simulink library "Linkage_Systems"  (R2024a)
settings: Solver=VariableStepAuto  StartTime=0.0  StopTime=10.0  RelTol=1e-3
undefined symbols (not defined in the file): Init, Vehicle
libraries: Linkage_DW_B x1, Linkage_DW_Pullrod x1, Linkage_DW_Pullrod_NoSteer x1, Linkage_DW_Pushrod x1, Linkage_DW_Pushrod_NoSteer x1, Linkage_DW_A x1, Linkage_Link5C_S2LAF x1, Linkage_Link5_S2LAC_AU_NoSteer x1, Linkage_Link5_S2LAF x1, Linkage_Link5_S2LAR x1, Linkage_MacPherson x1, Linkage_MacPherson_SpLA x1
(part 2 of 2)

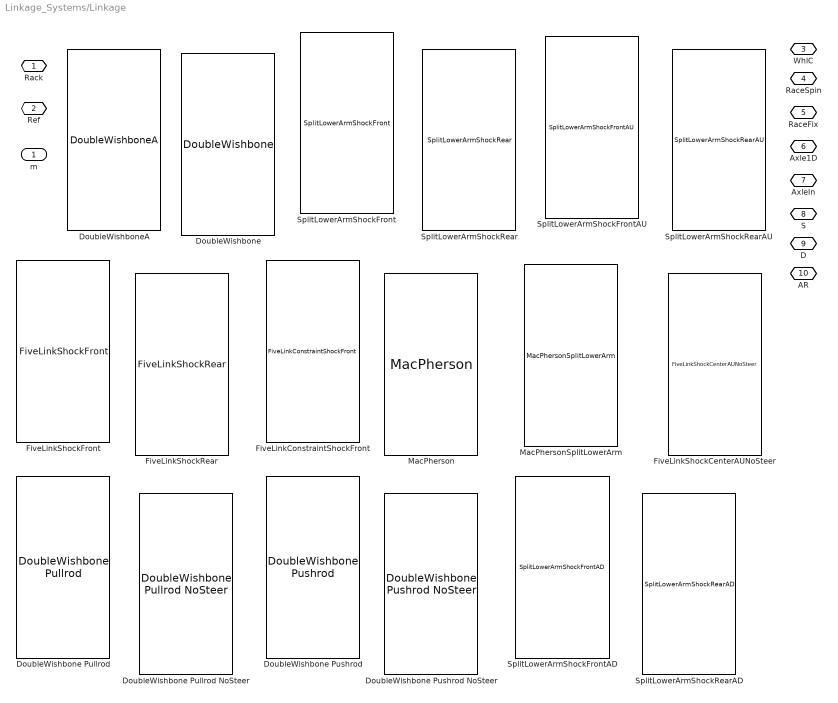
== system Linkage_Systems/Linkage ==
  DoubleWishbone : Linkage_DW_B/DoubleWishbone  VariantControl=DoubleWishbone  popup_leftRight=Left  hp_in_f_ua=Linkage.UpperWishbone.sInboardF.Value  hp_in_r_ua=Linkage.UpperWishbone.sInboardR.Value  hp_out_ua=Linkage.UpperWishbone.sOutboard.Value  hp_in_f_la=Linkage.LowerWishbone.sInboardF.Value  hp_in_r_la=Linkage.LowerWishbone.sInboardR.Value  hp_out_la=Linkage.LowerWishbone.sOutboard.Value  hp_arb=Linkage.LowerWishbone.sARB.Value  hp_upr_cg=Linkage.Upright.sCG.Value  hp_upr_wc=Linkage.Upright.sWheelCentre.Value  hp_in_rod=Linkage.TrackRod.sInboard.Value  hp_upr_rod=Linkage.TrackRod.sOutboard.Value  hp_spr_top=Linkage.Shock.sTop.Value  hp_spr_bot=Linkage.Shock.sBottom.Value  clr_hp=Visual.hp.clr  opc_hp=Visual.hp.opc  size_hp=Visual.hp.rad  Upper_Arm_to_Subframe=Linkage.Upper_Arm_to_Subframe  ua_mass=Linkage.UpperWishbone.m.Value  clr_ua=Visual.UpperArm.clr  opc_ua=Visual.part.opc  radius_ua=Visual.UpperArm.rad  Lower_Arm_to_Subframe=Linkage.Lower_Arm_to_Subframe  arm_mass=Linkage.LowerWishbone.m.Value  clr_la=Visual.LowerArm.clr  opc_la=Visual.part.opc  radius_la=Visual.LowerArm.rad  shock_pist_mass=Linkage.Shock.mPiston.Value  shock_cyl_mass=Linkage.Shock.mCylinder.Value  up_lim_bumpstop=Linkage.Endstop.xMax.Value  low_lim_bumpstop=Linkage.Endstop.xMin.Value  clr_conn_shock=Visual.hp.clr  opc_conn_shock=Visual.hp.opc  size_conn_shock=Visual.hp.rad  clr_shock_cyl=Visual.Shock.cyl.clr  opc_shock_cyl=Visual.part.opc  radius_shock_cyl=Visual.Shock.cyl.rad  clr_shock_piston=Visual.Shock.piston.clr  opc_shock_piston=Visual.part.opc  clr_shock_bumpstop=Visual.Shock.bumpstop.clr  opc_shock_bumpstop=Visual.part.opc  deadvol_len_shock_cyl=Visual.Shock.dead_length  piston_len_shock=Visual.Shock.piston.len  cyl_cap_len_shock=Visual.Shock.cap.len  bumpstop_len_shock=Visual.Shock.bumpstop.len  upr_mass=Linkage.Upright.m.Value  atoe=Linkage.Upright.aToe.Value  acamber=Linkage.Upright.aCamber.Value  axle_len=Linkage.Upright.xAxle.Value  axle_whlc_to_bearing=Linkage.Upright.xWCtoBearing.Value  axle_mass=Linkage.Upright.mAxle.Value  clr_conn_upr=Visual.hp.clr  opc_conn_upr=Visual.hp.opc  size_conn_upr=Visual.hp.rad  clr_upr=Visual.Upright.clr  opc_upr=Visual.part.opc  radius_upr=Visual.Upright.rad  clr_axle=Visual.Axle.clr  opc_axle=Visual.part.opc  radius_axle=Visual.Axle.rad  rod_mass=Linkage.TrackRod.m.Value  clr_conn_rod=Visual.hp.clr  opc_conn_rod=Visual.hp.opc  size_conn_rod=Visual.hp.rad  clr_rod=Visual.TrackRod.clr  opc_rod=Visual.part.opc  radius_rod=Visual.TrackRod.rad  whl_init_spd_lr=InitLinkage.nWheel.Value
  DoubleWishbone Pullrod : Linkage_DW_Pullrod/DoubleWishbone Pullrod  VariantControl=DoubleWishbonePullrod  popup_leftRight=Left  hp_in_f_ua=Linkage.UpperWishbone.sInboardF.Value  hp_in_r_ua=Linkage.UpperWishbone.sInboardR.Value  hp_out_ua=Linkage.UpperWishbone.sOutboard.Value  hp_in_f_la=Linkage.LowerWishbone.sInboardF.Value  hp_in_r_la=Linkage.LowerWishbone.sInboardR.Value  hp_out_la=Linkage.LowerWishbone.sOutboard.Value  hp_pullrod_out=Linkage.Pullrod.sUpperArm.Value  hp_pullrod_in=Linkage.Pullrod.sBellcrank.Value  hp_arb=Linkage.Bellcrank.sAntiRollBar.Value  hp_bcr_pivot=Linkage.Bellcrank.sPivot.Value  hp_upr_cg=Linkage.Upright.sCG.Value  hp_upr_wc=Linkage.Upright.sWheelCentre.Value  hp_in_rod=Linkage.TrackRod.sInboard.Value  hp_upr_rod=Linkage.TrackRod.sOutboard.Value  hp_spr_body=Linkage.Shock.sTop.Value  hp_spr_bcr=Linkage.Shock.sBottom.Value  clr_hp=Visual.hp.clr  opc_hp=Visual.hp.opc  size_hp=Visual.hp.rad  Upper_Arm_to_Subframe=Linkage.Upper_Arm_to_Subframe  ua_mass=Linkage.UpperWishbone.m.Value  clr_ua=Visual.UpperArm.clr  opc_ua=Visual.part.opc  radius_ua=Visual.UpperArm.rad  Lower_Arm_to_Subframe=Linkage.Lower_Arm_to_Subframe  la_mass=Linkage.LowerWishbone.m.Value  clr_la=Visual.LowerArm.clr  opc_la=Visual.part.opc  radius_la=Visual.LowerArm.rad  shock_pist_mass=Linkage.Shock.mPiston.Value  shock_cyl_mass=Linkage.Shock.mCylinder.Value  up_lim_bumpstop=Linkage.Endstop.xMax.Value  low_lim_bumpstop=Linkage.Endstop.xMin.Value  clr_conn_shock=Visual.hp.clr  opc_conn_shock=Visual.hp.opc  size_conn_shock=Visual.hp.rad  clr_shock_cyl=Visual.Shock.cyl.clr  opc_shock_cyl=Visual.part.opc  radius_shock_cyl=Visual.Shock.cyl.rad  clr_shock_piston=Visual.Shock.piston.clr  opc_shock_piston=Visual.part.opc  clr_shock_bumpstop=Visual.Shock.bumpstop.clr  opc_shock_bumpstop=Visual.part.opc  deadvol_len_shock_cyl=Visual.Shock.dead_length  piston_len_shock=Visual.Shock.piston.len  cyl_cap_len_shock=Visual.Shock.cap.len  bumpstop_len_shock=Visual.Shock.bumpstop.len  upr_mass=Linkage.Upright.m.Value  atoe=Linkage.Upright.aToe.Value  acamber=Linkage.Upright.aCamber.Value  axle_len=Linkage.Upright.xAxle.Value  axle_whlc_to_bearing=Linkage.Upright.xWCtoBearing.Value  axle_mass=Linkage.Upright.mAxle.Value  clr_conn_upr=Visual.hp.clr  opc_conn_upr=Visual.hp.opc  size_conn_upr=Visual.hp.rad  clr_upr=Visual.Upright.clr  opc_upr=Visual.part.opc  radius_upr=Visual.Upright.rad  clr_axle=Visual.Axle.clr  opc_axle=Visual.part.opc  radius_axle=Visual.Axle.rad  rod_mass=Linkage.TrackRod.m.Value  clr_conn_rod=Visual.hp.clr  opc_conn_rod=Visual.hp.opc  size_conn_rod=Visual.hp.rad  clr_rod=Visual.TrackRod.clr  opc_rod=Visual.part.opc  radius_rod=Visual.TrackRod.rad  bcr_mass=Linkage.Bellcrank.m.Value  clr_bcr=Visual.Bellcrank.clr  opc_bcr=Visual.part.opc  radius_bcr=Visual.Bellcrank.rad  pullrod_mass=Linkage.Pullrod.m.Value  clr_conn_pullrod=Visual.hp.clr  opc_conn_pullrod=Visual.hp.opc  size_conn_pullrod=Visual.hp.rad  clr_pullrod=Visual.Pullrod.clr  opc_pullrod=Visual.part.opc  radius_pullrod=Visual.Pullrod.rad  whl_init_spd_lr=InitLinkage.nWheel.Value
  DoubleWishbone Pullrod NoSteer : Linkage_DW_Pullrod_NoSteer/DoubleWishbone Pullrod NoSteer  VariantControl=DoubleWishbonePullrodNoSteer  popup_leftRight=Left  hp_in_f_ua=Linkage.UpperWishbone.sInboardF.Value  hp_in_r_ua=Linkage.UpperWishbone.sInboardR.Value  hp_out_ua=Linkage.UpperWishbone.sOutboard.Value  hp_in_f_la=Linkage.LowerWishbone.sInboardF.Value  hp_in_r_la=Linkage.LowerWishbone.sInboardR.Value  hp_out_la=Linkage.LowerWishbone.sOutboard.Value  hp_pullrod_out=Linkage.Pullrod.sUpperArm.Value  hp_pullrod_in=Linkage.Pullrod.sBellcrank.Value  hp_bcr_pivot=Linkage.Bellcrank.sPivot.Value  hp_arb=Linkage.Bellcrank.sAntiRollBar.Value  hp_upr_cg=Linkage.Upright.sCG.Value  hp_upr_wc=Linkage.Upright.sWheelCentre.Value  hp_upr_rod=Linkage.TrackRod.sOutboard.Value  hp_uar_rod=Linkage.TrackRod.sInboard.Value  hp_spr_body=Linkage.Shock.sTop.Value  hp_spr_bcr=Linkage.Shock.sBottom.Value  clr_hp=Visual.hp.clr  opc_hp=Visual.hp.opc  size_hp=Visual.hp.rad  Upper_Arm_to_Subframe=Linkage.Upper_Arm_to_Subframe  ua_mass=Linkage.UpperWishbone.m.Value  clr_ua=Visual.UpperArm.clr  opc_ua=Visual.part.opc  radius_ua=Visual.UpperArm.rad  Lower_Arm_to_Subframe=Linkage.Lower_Arm_to_Subframe  la_mass=Linkage.LowerWishbone.m.Value  clr_la=Visual.LowerArm.clr  opc_la=Visual.part.opc  radius_la=Visual.LowerArm.rad  shock_pist_mass=Linkage.Shock.mPiston.Value  shock_cyl_mass=Linkage.Shock.mCylinder.Value  up_lim_bumpstop=Linkage.Endstop.xMax.Value  low_lim_bumpstop=Linkage.Endstop.xMin.Value  clr_conn_shock=Visual.hp.clr  opc_conn_shock=Visual.hp.opc  size_conn_shock=Visual.hp.rad  clr_shock_cyl=Visual.Shock.cyl.clr  opc_shock_cyl=Visual.part.opc  radius_shock_cyl=Visual.Shock.cyl.rad  clr_shock_piston=Visual.Shock.piston.clr  opc_shock_piston=Visual.part.opc  clr_shock_bumpstop=Visual.Shock.bumpstop.clr  opc_shock_bumpstop=Visual.part.opc  deadvol_len_shock_cyl=Visual.Shock.dead_length  piston_len_shock=Visual.Shock.piston.len  cyl_cap_len_shock=Visual.Shock.cap.len  bumpstop_len_shock=Visual.Shock.bumpstop.len  upr_mass=Linkage.Upright.m.Value  atoe=Linkage.Upright.aToe.Value  acamber=Linkage.Upright.aCamber.Value  axle_len=Linkage.Upright.xAxle.Value  axle_whlc_to_bearing=Linkage.Upright.xWCtoBearing.Value  axle_mass=Linkage.Upright.mAxle.Value  clr_conn_upr=Visual.hp.clr  opc_conn_upr=Visual.hp.opc  size_conn_upr=Visual.hp.rad  clr_upr=Visual.Upright.clr  opc_upr=Visual.part.opc  radius_upr=Visual.Upright.rad  clr_axle=Visual.Axle.clr  opc_axle=Visual.part.opc  radius_axle=Visual.Axle.rad  rod_mass=Linkage.TrackRod.m.Value  clr_conn_rod=Visual.hp.clr  opc_conn_rod=Visual.hp.opc  size_conn_rod=Visual.hp.rad  clr_rod=Visual.TrackRod.clr  opc_rod=Visual.part.opc  radius_rod=Visual.TrackRod.rad  bcr_mass=Linkage.Bellcrank.m.Value  clr_bcr=Visual.Bellcrank.clr  opc_bcr=Visual.part.opc  radius_bcr=Visual.Bellcrank.rad  pullrod_mass=Linkage.Pullrod.m.Value  clr_conn_pullrod=Visual.hp.clr  opc_conn_pullrod=Visual.hp.opc  size_conn_pullrod=Visual.hp.rad  clr_pullrod=Visual.Pullrod.clr  opc_pullrod=Visual.part.opc  radius_pullrod=Visual.Pullrod.rad  whl_init_spd_lr=InitLinkage.nWheel.Value
  DoubleWishbone Pushrod : Linkage_DW_Pushrod/DoubleWishbone Pushrod  VariantControl=DoubleWishbonePushrod  popup_leftRight=Left  hp_in_f_ua=Linkage.UpperWishbone.sInboardF.Value  hp_in_r_ua=Linkage.UpperWishbone.sInboardR.Value  hp_out_ua=Linkage.UpperWishbone.sOutboard.Value  hp_in_f_la=Linkage.LowerWishbone.sInboardF.Value  hp_in_r_la=Linkage.LowerWishbone.sInboardR.Value  hp_out_la=Linkage.LowerWishbone.sOutboard.Value  hp_pushrod_out=Linkage.Pushrod.sLowerArm.Value  hp_pushrod_in=Linkage.Pushrod.sBellcrank.Value  hp_arb=Linkage.Bellcrank.sAntiRollBar.Value  hp_bcr_pivot=Linkage.Bellcrank.sPivot.Value  hp_upr_cg=Linkage.Upright.sCG.Value  hp_upr_wc=Linkage.Upright.sWheelCentre.Value  hp_in_rod=Linkage.TrackRod.sInboard.Value  hp_upr_rod=Linkage.TrackRod.sOutboard.Value  hp_spr_body=Linkage.Shock.sTop.Value  hp_spr_bcr=Linkage.Shock.sBottom.Value  clr_hp=Visual.hp.clr  opc_hp=Visual.hp.opc  size_hp=Visual.hp.rad  Upper_Arm_to_Subframe=Linkage.Upper_Arm_to_Subframe  ua_mass=Linkage.UpperWishbone.m.Value  clr_ua=Visual.UpperArm.clr  opc_ua=Visual.part.opc  radius_ua=Visual.UpperArm.rad  Lower_Arm_to_Subframe=Linkage.Lower_Arm_to_Subframe  la_mass=Linkage.LowerWishbone.m.Value  clr_la=Visual.LowerArm.clr  opc_la=Visual.part.opc  radius_la=Visual.LowerArm.rad  shock_pist_mass=Linkage.Shock.mPiston.Value  shock_cyl_mass=Linkage.Shock.mCylinder.Value  up_lim_bumpstop=Linkage.Endstop.xMax.Value  low_lim_bumpstop=Linkage.Endstop.xMin.Value  clr_conn_shock=Visual.hp.clr  opc_conn_shock=Visual.hp.opc  size_conn_shock=Visual.hp.rad  clr_shock_cyl=Visual.Shock.cyl.clr  opc_shock_cyl=Visual.part.opc  radius_shock_cyl=Visual.Shock.cyl.rad  clr_shock_piston=Visual.Shock.piston.clr  opc_shock_piston=Visual.part.opc  clr_shock_bumpstop=Visual.Shock.bumpstop.clr  opc_shock_bumpstop=Visual.part.opc  deadvol_len_shock_cyl=Visual.Shock.dead_length  piston_len_shock=Visual.Shock.piston.len  cyl_cap_len_shock=Visual.Shock.cap.len  bumpstop_len_shock=Visual.Shock.bumpstop.len  upr_mass=Linkage.Upright.m.Value  atoe=Linkage.Upright.aToe.Value  acamber=Linkage.Upright.aCamber.Value  axle_len=Linkage.Upright.xAxle.Value  axle_whlc_to_bearing=Linkage.Upright.xWCtoBearing.Value  axle_mass=Linkage.Upright.mAxle.Value  clr_conn_upr=Visual.hp.clr  opc_conn_upr=Visual.hp.opc  size_conn_upr=Visual.hp.rad  clr_upr=Visual.Upright.clr  opc_upr=Visual.part.opc  radius_upr=Visual.Upright.rad  clr_axle=Visual.Axle.clr  opc_axle=Visual.part.opc  radius_axle=Visual.Axle.rad  rod_mass=Linkage.TrackRod.m.Value  clr_conn_rod=Visual.hp.clr  opc_conn_rod=Visual.hp.opc  size_conn_rod=Visual.hp.rad  clr_rod=Visual.TrackRod.clr  opc_rod=Visual.part.opc  radius_rod=Visual.TrackRod.rad  bcr_mass=Linkage.Bellcrank.m.Value  clr_bcr=Visual.Bellcrank.clr  opc_bcr=Visual.part.opc  radius_bcr=Visual.Bellcrank.rad  pushrod_mass=Linkage.Pushrod.m.Value  clr_conn_pushrod=Visual.hp.clr  opc_conn_pushrod=Visual.hp.opc  size_conn_pushrod=Visual.hp.rad  clr_pushrod=Visual.Pushrod.clr  opc_pushrod=Visual.part.opc  radius_pushrod=Visual.Pushrod.rad  whl_init_spd_lr=InitLinkage.nWheel.Value
  DoubleWishbone Pushrod NoSteer : Linkage_DW_Pushrod_NoSteer/DoubleWishbone Pushrod NoSteer  VariantControl=DoubleWishbonePushrodNoSteer  popup_leftRight=Left  hp_in_f_ua=Linkage.UpperWishbone.sInboardF.Value  hp_in_r_ua=Linkage.UpperWishbone.sInboardR.Value  hp_out_ua=Linkage.UpperWishbone.sOutboard.Value  hp_in_f_la=Linkage.LowerWishbone.sInboardF.Value  hp_in_r_la=Linkage.LowerWishbone.sInboardR.Value  hp_out_la=Linkage.LowerWishbone.sOutboard.Value  hp_pushrod_out=Linkage.Pushrod.sLowerArm.Value  hp_pushrod_in=Linkage.Pushrod.sBellcrank.Value  hp_arb=Linkage.Bellcrank.sAntiRollBar.Value  hp_bcr_pivot=Linkage.Bellcrank.sPivot.Value  hp_upr_cg=Linkage.Upright.sCG.Value  hp_upr_wc=Linkage.Upright.sWheelCentre.Value  hp_track_in=Linkage.TrackRod.sInboard.Value  hp_track_out=Linkage.TrackRod.sOutboard.Value  hp_spr_body=Linkage.Shock.sTop.Value  hp_spr_bcr=Linkage.Shock.sBottom.Value  clr_hp=Visual.hp.clr  opc_hp=Visual.hp.opc  size_hp=Visual.hp.rad  Upper_Arm_to_Subframe=Linkage.Upper_Arm_to_Subframe  ua_mass=Linkage.UpperWishbone.m.Value  clr_ua=Visual.UpperArm.clr  opc_ua=Visual.part.opc  radius_ua=Visual.UpperArm.rad  Lower_Arm_to_Subframe=Linkage.Lower_Arm_to_Subframe  la_mass=Linkage.LowerWishbone.m.Value  clr_la=Visual.LowerArm.clr  opc_la=Visual.part.opc  radius_la=Visual.LowerArm.rad  shock_pist_mass=Linkage.Shock.mPiston.Value  shock_cyl_mass=Linkage.Shock.mCylinder.Value  up_lim_bumpstop=Linkage.Endstop.xMax.Value  low_lim_bumpstop=Linkage.Endstop.xMin.Value  clr_conn_shock=Visual.hp.clr  opc_conn_shock=Visual.hp.opc  size_conn_shock=Visual.hp.rad  clr_shock_cyl=Visual.Shock.cyl.clr  opc_shock_cyl=Visual.part.opc  radius_shock_cyl=Visual.Shock.cyl.rad  clr_shock_piston=Visual.Shock.piston.clr  opc_shock_piston=Visual.part.opc  clr_shock_bumpstop=Visual.Shock.bumpstop.clr  opc_shock_bumpstop=Visual.part.opc  deadvol_len_shock_cyl=Visual.Shock.dead_length  piston_len_shock=Visual.Shock.piston.len  cyl_cap_len_shock=Visual.Shock.cap.len  bumpstop_len_shock=Visual.Shock.bumpstop.len  upr_mass=Linkage.Upright.m.Value  atoe=Linkage.Upright.aToe.Value  acamber=Linkage.Upright.aCamber.Value  axle_len=Linkage.Upright.xAxle.Value  axle_whlc_to_bearing=Linkage.Upright.xWCtoBearing.Value  axle_mass=Linkage.Upright.mAxle.Value  clr_conn_upr=Visual.hp.clr  opc_conn_upr=Visual.hp.opc  size_conn_upr=Visual.hp.rad  clr_upr=Visual.Upright.clr  opc_upr=Visual.part.opc  radius_upr=Visual.Upright.rad  clr_axle=Visual.Axle.clr  opc_axle=Visual.part.opc  radius_axle=Visual.Axle.rad  rod_mass=Linkage.TrackRod.m.Value  clr_conn_rod=Visual.hp.clr  opc_conn_rod=Visual.hp.opc  size_conn_rod=Visual.hp.rad  clr_rod=Visual.TrackRod.clr  opc_rod=Visual.part.opc  radius_rod=Visual.TrackRod.rad  bcr_mass=Linkage.Bellcrank.m.Value  clr_bcr=Visual.Bellcrank.clr  opc_bcr=Visual.part.opc  radius_bcr=Visual.Bellcrank.rad  pushrod_mass=Linkage.Pushrod.m.Value  clr_conn_pushrod=Visual.hp.clr  opc_conn_pushrod=Visual.hp.opc  size_conn_pushrod=Visual.hp.rad  clr_pushrod=Visual.Pushrod.clr  opc_pushrod=Visual.part.opc  radius_pushrod=Visual.Pushrod.rad  whl_init_spd_lr=InitLinkage.nWheel.Value
  DoubleWishboneA : Linkage_DW_A/DoubleWishboneA  VariantControl=DoubleWishboneA  popup_leftRight=Left  hp_in_f_ua=Linkage.UpperWishbone.sInboardF.Value  hp_in_r_ua=Linkage.UpperWishbone.sInboardR.Value  hp_out_ua=Linkage.UpperWishbone.sOutboard.Value  hp_in_f_la=Linkage.LowerWishbone.sInboardF.Value  hp_in_r_la=Linkage.LowerWishbone.sInboardR.Value  hp_out_la=Linkage.LowerWishbone.sOutboard.Value  hp_arb=Linkage.LowerWishbone.sARB.Value  hp_upr_cg=Linkage.Upright.sCG.Value  hp_upr_wc=Linkage.Upright.sWheelCentre.Value  hp_in_rod=Linkage.TrackRod.sInboard.Value  hp_upr_rod=Linkage.TrackRod.sOutboard.Value  hp_spr_top=Linkage.Shock.sTop.Value  hp_spr_bot=Linkage.Shock.sBottom.Value  clr_hp=Visual.hp.clr  opc_hp=Visual.hp.opc  size_hp=Visual.hp.rad  Upper_Arm_to_Subframe=Linkage.Upper_Arm_to_Subframe  ua_mass=Linkage.UpperWishbone.m.Value  clr_ua=Visual.UpperArm.clr  opc_ua=Visual.part.opc  radius_ua=Visual.UpperArm.rad  Lower_Arm_to_Subframe=Linkage.Lower_Arm_to_Subframe  la_mass=Linkage.LowerWishbone.m.Value  clr_la=Visual.LowerArm.clr  opc_la=Visual.part.opc  radius_la=Visual.LowerArm.rad  shock_pist_mass=Linkage.Shock.mPiston.Value  shock_cyl_mass=Linkage.Shock.mCylinder.Value  up_lim_bumpstop=Linkage.Endstop.xMax.Value  low_lim_bumpstop=Linkage.Endstop.xMin.Value  clr_conn_shock=Visual.hp.clr  opc_conn_shock=Visual.hp.opc  size_conn_shock=Visual.hp.rad  clr_shock_cyl=Visual.Shock.cyl.clr  opc_shock_cyl=Visual.part.opc  radius_shock_cyl=Visual.Shock.cyl.rad  clr_shock_piston=Visual.Shock.piston.clr  opc_shock_piston=Visual.part.opc  clr_shock_bumpstop=Visual.Shock.bumpstop.clr  opc_shock_bumpstop=Visual.part.opc  deadvol_len_shock_cyl=Visual.Shock.dead_length  piston_len_shock=Visual.Shock.piston.len  cyl_cap_len_shock=Visual.Shock.cap.len  bumpstop_len_shock=Visual.Shock.bumpstop.len  atoe=Linkage.Upright.aToe.Value  acamber=Linkage.Upright.aCamber.Value  upr_mass=Linkage.Upright.m.Value  axle_len=Linkage.Upright.xAxle.Value  axle_whlc_to_bearing=Linkage.Upright.xWCtoBearing.Value  axle_mass=Linkage.Upright.mAxle.Value  clr_conn_upr=Visual.hp.clr  opc_conn_upr=Visual.hp.opc  size_conn_upr=Visual.hp.rad  clr_upr=Visual.Upright.clr  opc_upr=Visual.part.opc  radius_upr=Visual.Upright.rad  clr_axle=Visual.Axle.clr  opc_axle=Visual.part.opc  radius_axle=Visual.Axle.rad  steer_class=Linkage.Steer.class.Value  rod_mass=Linkage.TrackRod.m.Value  clr_conn_rod=Visual.hp.clr  opc_conn_rod=Visual.hp.opc  size_conn_rod=Visual.hp.rad  clr_rod_str=Visual.SteeringArm.clr  opc_rod_str=Visual.part.opc  radius_rod_str=Visual.SteeringArm.rad  clr_rod=Visual.TrackRod.clr  opc_rod=Visual.part.opc  radius_rod=Visual.TrackRod.rad  whl_init_spd_lr=InitLinkage.nWheel.Value
  FiveLinkConstraintShockFront : Linkage_Link5C_S2LAF/FiveLinkConstraintShockFront  VariantControl=FiveLinkConstraintShockFront  popup_leftRight=Left  hp_in_f_ua=Linkage.UpperArmF.sInboard.Value  hp_in_r_ua=Linkage.UpperArmR.sInboard.Value  hp_out_f_ua=Linkage.UpperArmF.sOutboard.Value  hp_out_r_ua=Linkage.UpperArmR.sOutboard.Value  hp_in_f_la=Linkage.LowerArmF.sInboard.Value  hp_in_r_la=Linkage.LowerArmR.sInboard.Value  hp_out_f_la=Linkage.LowerArmF.sOutboard.Value  hp_out_r_la=Linkage.LowerArmR.sOutboard.Value  hp_arb=Linkage.LowerArmR.sARB.Value  hp_upr_cg=Linkage.Upright.sCG.Value  hp_upr_wc=Linkage.Upright.sWheelCentre.Value  hp_in_rod=Linkage.TrackRod.sInboard.Value  hp_upr_rod=Linkage.TrackRod.sOutboard.Value  hp_spr_top=Linkage.Shock.sTop.Value  hp_spr_bot=Linkage.Shock.sBottom.Value  clr_hp=Visual.hp.clr  opc_hp=Visual.hp.opc  size_hp=Visual.hp.rad  uaf_mass=Linkage.UpperArmF.m.Value  uar_mass=Linkage.UpperArmR.m.Value  laf_mass=Linkage.LowerArmF.m.Value  lar_mass=Linkage.LowerArmR.m.Value  clr_conn_links=Visual.hp.clr  opc_conn_links=Visual.hp.opc  size_conn_links=Visual.hp.rad  clr_uaf=Visual.UpperArm.clr  opc_uaf=Visual.part.opc  radius_uaf=Visual.UpperArm.rad  clr_uar=Visual.UpperArm.clr  opc_uar=Visual.part.opc  radius_uar=Visual.UpperArm.rad  clr_laf=Visual.LowerArm.clr  opc_laf=Visual.part.opc  radius_laf=Visual.LowerArm.rad  clr_lar=Visual.LowerArm.clr  opc_lar=Visual.part.opc  radius_lar=Visual.LowerArm.rad  shock_pist_mass=Linkage.Shock.mPiston.Value  shock_cyl_mass=Linkage.Shock.mCylinder.Value  up_lim_bumpstop=Linkage.Endstop.xMax.Value  low_lim_bumpstop=Linkage.Endstop.xMin.Value  clr_conn_shock=Visual.hp.clr  opc_conn_shock=Visual.hp.opc  size_conn_shock=Visual.hp.rad  clr_shock_cyl=Visual.Shock.cyl.clr  opc_shock_cyl=Visual.part.opc  radius_shock_cyl=Visual.Shock.cyl.rad  clr_shock_piston=Visual.Shock.piston.clr  opc_shock_piston=Visual.part.opc  clr_shock_bumpstop=Visual.Shock.bumpstop.clr  opc_shock_bumpstop=Visual.part.opc  deadvol_len_shock_cyl=Visual.Shock.dead_length  piston_len_shock=Visual.Shock.piston.len  cyl_cap_len_shock=Visual.Shock.cap.len  bumpstop_len_shock=Visual.Shock.bumpstop.len  atoe=Linkage.Upright.aToe.Value  acamber=Linkage.Upright.aCamber.Value  upr_mass=Linkage.Upright.m.Value  axle_len=Linkage.Upright.xAxle.Value  axle_whlc_to_bearing=Linkage.Upright.xWCtoBearing.Value  axle_mass=Linkage.Upright.mAxle.Value  clr_conn_upr=Visual.hp.clr  opc_conn_upr=Visual.hp.opc  size_conn_upr=Visual.hp.rad  clr_upr=Visual.Upright.clr  opc_upr=Visual.part.opc  radius_upr=Visual.Upright.rad  clr_axle=Visual.Axle.clr  opc_axle=Visual.part.opc  radius_axle=Visual.Axle.rad  rod_mass=Linkage.TrackRod.m.Value  clr_conn_rod=Visual.hp.clr  opc_conn_rod=Visual.hp.opc  size_conn_rod=Visual.hp.rad  clr_rod=Visual.TrackRod.clr  opc_rod=Visual.part.opc  radius_rod=Visual.TrackRod.rad  whl_init_spd_lr=InitLinkage.nWheel.Value
  FiveLinkShockCenterAUNoSteer : Linkage_Link5_S2LAC_AU_NoSteer/FiveLinkShockCenterAUNoSteer  VariantControl=FiveLinkShockCenterAUNoSteer  popup_leftRight=Left  hp_in_f_ua=Linkage.UpperArmF.sInboard.Value  hp_in_r_ua=Linkage.UpperArmR.sInboard.Value  hp_out_f_ua=Linkage.UpperArmF.sOutboard.Value  hp_out_r_ua=Linkage.UpperArmR.sOutboard.Value  hp_in_f_la=Linkage.LowerArmF.sInboard.Value  hp_in_c_la=Linkage.LowerArmC.sInboard.Value  hp_in_r_la=Linkage.LowerArmR.sInboard.Value  hp_out_f_la=Linkage.LowerArmF.sOutboard.Value  hp_out_c_la=Linkage.LowerArmC.sOutboard.Value  hp_out_r_la=Linkage.LowerArmR.sOutboard.Value  hp_arb=Linkage.Upright.sARB.Value  hp_upr_cg=Linkage.Upright.sCG.Value  hp_upr_wc=Linkage.Upright.sWheelCentre.Value  hp_spr_top=Linkage.Shock.sTop.Value  hp_spr_bot=Linkage.Shock.sBottom.Value  clr_hp=Visual.hp.clr  opc_hp=Visual.hp.opc  size_hp=Visual.hp.rad  UpperArmF_to_Subframe=Linkage.UpperArmF_to_Subframe  UpperArmR_to_Subframe=Linkage.UpperArmR_to_Subframe  LowerArmF_to_Subframe=Linkage.LowerArmF_to_Subframe  LowerArmC_to_Subframe=Linkage.LowerArmC_to_Subframe  LowerArmR_to_Subframe=Linkage.LowerArmR_to_Subframe  UpperArmF_to_Upright=Linkage.UpperArmF_to_Upright  UpperArmR_to_Upright=Linkage.UpperArmR_to_Upright  LowerArmF_to_Upright=Linkage.LowerArmF_to_Upright  LowerArmC_to_Upright=Linkage.LowerArmC_to_Upright  LowerArmR_to_Upright=Linkage.LowerArmR_to_Upright  uaf_mass=Linkage.UpperArmF.m.Value  uar_mass=Linkage.UpperArmR.m.Value  laf_mass=Linkage.LowerArmF.m.Value  lac_mass=Linkage.LowerArmC.m.Value  lar_mass=Linkage.LowerArmR.m.Value  clr_conn_rod=Visual.hp.clr  opc_conn_rod=Visual.hp.opc  size_conn_rod=Visual.hp.rad  clr_uaf=Visual.UpperArm.clr  opc_uaf=Visual.part.opc  radius_uaf=Visual.UpperArm.rad  clr_uar=Visual.UpperArm.clr  opc_uar=Visual.part.opc  radius_uar=Visual.UpperArm.rad  clr_laf=Visual.LowerArm.clr  opc_laf=Visual.part.opc  radius_laf=Visual.LowerArm.rad  clr_lac=Visual.LowerArm.clr  opc_lac=Visual.part.opc  radius_lac=Visual.LowerArm.rad  clr_lar=Visual.LowerArm.clr  opc_lar=Visual.part.opc  radius_lar=Visual.LowerArm.rad  shock_pist_mass=Linkage.Shock.mPiston.Value  shock_cyl_mass=Linkage.Shock.mCylinder.Value  up_lim_bumpstop=Linkage.Endstop.xMax.Value  low_lim_bumpstop=Linkage.Endstop.xMin.Value  clr_conn_shock=Visual.hp.clr  opc_conn_shock=Visual.hp.opc  size_conn_shock=Visual.hp.rad  clr_shock_cyl=Visual.Shock.cyl.clr  opc_shock_cyl=Visual.part.opc  radius_shock_cyl=Visual.Shock.cyl.rad  clr_shock_piston=Visual.Shock.piston.clr  opc_shock_piston=Visual.part.opc  clr_shock_bumpstop=Visual.Shock.bumpstop.clr  opc_shock_bumpstop=Visual.part.opc  deadvol_len_shock_cyl=Visual.Shock.dead_length  piston_len_shock=Visual.Shock.piston.len  cyl_cap_len_shock=Visual.Shock.cap.len  bumpstop_len_shock=Visual.Shock.bumpstop.len  atoe=Linkage.Upright.aToe.Value  acamber=Linkage.Upright.aCamber.Value  upr_mass=Linkage.Upright.m.Value  axle_len=Linkage.Upright.xAxle.Value  axle_whlc_to_bearing=Linkage.Upright.xWCtoBearing.Value  axle_mass=Linkage.Upright.mAxle.Value  clr_conn_upr=Visual.hp.clr  opc_conn_upr=Visual.hp.opc  size_conn_upr=Visual.hp.rad  clr_upr=Visual.Upright.clr  opc_upr=Visual.part.opc  radius_upr=Visual.Upright.rad  clr_axle=Visual.Axle.clr  opc_axle=Visual.part.opc  radius_axle=Visual.Axle.rad  whl_init_spd_lr=InitLinkage.nWheel.Value
  FiveLinkShockFront : Linkage_Link5_S2LAF/FiveLinkShockFront  VariantControl=FiveLinkShockFront  popup_leftRight=Left  hp_in_f_ua=Linkage.UpperArmF.sInboard.Value  hp_in_r_ua=Linkage.UpperArmR.sInboard.Value  hp_out_f_ua=Linkage.UpperArmF.sOutboard.Value  hp_out_r_ua=Linkage.UpperArmR.sOutboard.Value  hp_in_f_la=Linkage.LowerArmF.sInboard.Value  hp_in_r_la=Linkage.LowerArmR.sInboard.Value  hp_out_f_la=Linkage.LowerArmF.sOutboard.Value  hp_out_r_la=Linkage.LowerArmR.sOutboard.Value  hp_arb=Linkage.LowerArmR.sARB.Value  hp_upr_cg=Linkage.Upright.sCG.Value  hp_upr_wc=Linkage.Upright.sWheelCentre.Value  hp_in_rod=Linkage.TrackRod.sInboard.Value  hp_upr_rod=Linkage.TrackRod.sOutboard.Value  hp_spr_top=Linkage.Shock.sTop.Value  hp_spr_bot=Linkage.Shock.sBottom.Value  clr_hp=Visual.hp.clr  opc_hp=Visual.hp.opc  size_hp=Visual.hp.rad  UpperArmF_to_Subframe=Linkage.UpperArmF_to_Subframe  UpperArmR_to_Subframe=Linkage.UpperArmR_to_Subframe  LowerArmF_to_Subframe=Linkage.LowerArmF_to_Subframe  LowerArmR_to_Subframe=Linkage.LowerArmR_to_Subframe  uaf_mass=Linkage.UpperArmF.m.Value  uar_mass=Linkage.UpperArmR.m.Value  laf_mass=Linkage.LowerArmF.m.Value  lar_mass=Linkage.LowerArmR.m.Value  clr_conn_links=Visual.hp.clr  opc_conn_links=Visual.hp.opc  size_conn_links=Visual.hp.rad  clr_uaf=Visual.UpperArm.clr  opc_uaf=Visual.part.opc  radius_uaf=Visual.UpperArm.rad  clr_uar=Visual.UpperArm.clr  opc_uar=Visual.part.opc  radius_uar=Visual.UpperArm.rad  clr_laf=Visual.LowerArm.clr  opc_laf=Visual.part.opc  radius_laf=Visual.LowerArm.rad  clr_lar=Visual.LowerArm.clr  opc_lar=Visual.part.opc  radius_lar=Visual.LowerArm.rad  shock_pist_mass=Linkage.Shock.mPiston.Value  shock_cyl_mass=Linkage.Shock.mCylinder.Value  up_lim_bumpstop=Linkage.Endstop.xMax.Value  low_lim_bumpstop=Linkage.Endstop.xMin.Value  clr_conn_shock=Visual.hp.clr  opc_conn_shock=Visual.hp.opc  size_conn_shock=Visual.hp.rad  clr_shock_cyl=Visual.Shock.cyl.clr  opc_shock_cyl=Visual.part.opc  radius_shock_cyl=Visual.Shock.cyl.rad  clr_shock_piston=Visual.Shock.piston.clr  opc_shock_piston=Visual.part.opc  clr_shock_bumpstop=Visual.Shock.bumpstop.clr  opc_shock_bumpstop=Visual.part.opc  deadvol_len_shock_cyl=Visual.Shock.dead_length  piston_len_shock=Visual.Shock.piston.len  cyl_cap_len_shock=Visual.Shock.cap.len  bumpstop_len_shock=Visual.Shock.bumpstop.len  atoe=Linkage.Upright.aToe.Value  acamber=Linkage.Upright.aCamber.Value  upr_mass=Linkage.Upright.m.Value  axle_len=Linkage.Upright.xAxle.Value  axle_whlc_to_bearing=Linkage.Upright.xWCtoBearing.Value  axle_mass=Linkage.Upright.mAxle.Value  clr_conn_upr=Visual.hp.clr  opc_conn_upr=Visual.hp.opc  size_conn_upr=Visual.hp.rad  clr_upr=Visual.Upright.clr  opc_upr=Visual.part.opc  radius_upr=Visual.Upright.rad  clr_axle=Visual.Axle.clr  opc_axle=Visual.part.opc  radius_axle=Visual.Axle.rad  rod_mass=Linkage.TrackRod.m.Value  clr_conn_rod=Visual.hp.clr  opc_conn_rod=Visual.hp.opc  size_conn_rod=Visual.hp.rad  clr_rod=Visual.TrackRod.clr  opc_rod=Visual.part.opc  radius_rod=Visual.TrackRod.rad  whl_init_spd_lr=InitLinkage.nWheel.Value
  FiveLinkShockRear : Linkage_Link5_S2LAR/FiveLinkShockRear  VariantControl=FiveLinkShockRear  popup_leftRight=Left  hp_in_f_ua=Linkage.UpperArmF.sInboard.Value  hp_in_r_ua=Linkage.UpperArmR.sInboard.Value  hp_out_f_ua=Linkage.UpperArmF.sOutboard.Value  hp_out_r_ua=Linkage.UpperArmR.sOutboard.Value  hp_in_f_la=Linkage.LowerArmF.sInboard.Value  hp_in_r_la=Linkage.LowerArmR.sInboard.Value  hp_out_f_la=Linkage.LowerArmF.sOutboard.Value  hp_out_r_la=Linkage.LowerArmR.sOutboard.Value  hp_arb=Linkage.LowerArmR.sARB.Value  hp_upr_cg=Linkage.Upright.sCG.Value  hp_upr_wc=Linkage.Upright.sWheelCentre.Value  hp_in_rod=Linkage.TrackRod.sInboard.Value  hp_upr_rod=Linkage.TrackRod.sOutboard.Value  hp_spr_top=Linkage.Shock.sTop.Value  hp_spr_bot=Linkage.Shock.sBottom.Value  clr_hp=Visual.hp.clr  opc_hp=Visual.hp.opc  size_hp=Visual.hp.rad  UpperArmF_to_Subframe=Linkage.UpperArmF_to_Subframe  UpperArmR_to_Subframe=Linkage.UpperArmR_to_Subframe  LowerArmF_to_Subframe=Linkage.LowerArmF_to_Subframe  LowerArmR_to_Subframe=Linkage.LowerArmR_to_Subframe  uaf_mass=Linkage.UpperArmF.m.Value  uar_mass=Linkage.UpperArmR.m.Value  laf_mass=Linkage.LowerArmF.m.Value  lar_mass=Linkage.LowerArmR.m.Value  clr_conn_links=Visual.hp.clr  opc_conn_links=Visual.hp.opc  size_conn_links=Visual.hp.rad  clr_uaf=Visual.UpperArm.clr  opc_uaf=Visual.part.opc  radius_uaf=Visual.UpperArm.rad  clr_uar=Visual.UpperArm.clr  opc_uar=Visual.part.opc  radius_uar=Visual.UpperArm.rad  clr_laf=Visual.LowerArm.clr  opc_laf=Visual.part.opc  radius_laf=Visual.LowerArm.rad  clr_lar=Visual.LowerArm.clr  opc_lar=Visual.part.opc  radius_lar=Visual.LowerArm.rad  shock_pist_mass=Linkage.Shock.mPiston.Value  shock_cyl_mass=Linkage.Shock.mCylinder.Value  up_lim_bumpstop=Linkage.Endstop.xMax.Value  low_lim_bumpstop=Linkage.Endstop.xMin.Value  clr_conn_shock=Visual.hp.clr  opc_conn_shock=Visual.hp.opc  size_conn_shock=Visual.hp.rad  clr_shock_cyl=Visual.Shock.cyl.clr  opc_shock_cyl=Visual.part.opc  radius_shock_cyl=Visual.Shock.cyl.rad  clr_shock_piston=Visual.Shock.piston.clr  opc_shock_piston=Visual.part.opc  clr_shock_bumpstop=Visual.Shock.bumpstop.clr  opc_shock_bumpstop=Visual.part.opc  deadvol_len_shock_cyl=Visual.Shock.dead_length  piston_len_shock=Visual.Shock.piston.len  cyl_cap_len_shock=Visual.Shock.cap.len  bumpstop_len_shock=Visual.Shock.bumpstop.len  atoe=Linkage.Upright.aToe.Value  acamber=Linkage.Upright.aCamber.Value  upr_mass=Linkage.Upright.m.Value  axle_len=Linkage.Upright.xAxle.Value  axle_whlc_to_bearing=Linkage.Upright.xWCtoBearing.Value  axle_mass=Linkage.Upright.mAxle.Value  clr_conn_upr=Visual.hp.clr  opc_conn_upr=Visual.hp.opc  size_conn_upr=Visual.hp.rad  clr_upr=Visual.Upright.clr  opc_upr=Visual.part.opc  radius_upr=Visual.Upright.rad  clr_axle=Visual.Axle.clr  opc_axle=Visual.part.opc  radius_axle=Visual.Axle.rad  rod_mass=Linkage.TrackRod.m.Value  clr_conn_rod=Visual.hp.clr  opc_conn_rod=Visual.hp.opc  size_conn_rod=Visual.hp.rad  clr_rod=Visual.TrackRod.clr  opc_rod=Visual.part.opc  radius_rod=Visual.TrackRod.rad  whl_init_spd_lr=InitLinkage.nWheel.Value
  MacPherson : Linkage_MacPherson/MacPherson  VariantControl=MacPherson  popup_leftRight=Left  hp_in_f_la=Linkage.LowerWishbone.sInboardF.Value  hp_in_r_la=Linkage.LowerWishbone.sInboardR.Value  hp_out_la=Linkage.LowerWishbone.sOutboard.Value  hp_upr_cg=Linkage.Upright.sCG.Value  hp_upr_wc=Linkage.Upright.sWheelCentre.Value  hp_upr_arb=Linkage.Upright.sARB.Value  hp_in_rod=Linkage.TrackRod.sInboard.Value  hp_upr_rod=Linkage.TrackRod.sOutboard.Value  hp_spr_top=Linkage.Shock.sTop.Value  hp_spr_bot=Linkage.Shock.sBottom.Value  clr_hp=Visual.hp.clr  opc_hp=Visual.hp.opc  size_hp=Visual.hp.rad  Lower_Arm_to_Subframe=Linkage.Lower_Arm_to_Subframe  la_mass=Linkage.LowerWishbone.m.Value  clr_la=Visual.LowerArm.clr  opc_la=Visual.part.opc  radius_la=Visual.LowerArm.rad  Shock_to_Subframe=Linkage.Shock_to_Subframe  shock_pist_mass=Linkage.Shock.mPiston.Value  shock_cyl_mass=Linkage.Shock.mCylinder.Value  up_lim_bumpstop=Linkage.Endstop.xMax.Value  low_lim_bumpstop=Linkage.Endstop.xMin.Value  clr_conn_shock=Visual.hp.clr  opc_conn_shock=Visual.hp.opc  size_conn_shock=Visual.hp.rad  clr_shock_cyl=Visual.Shock.cyl.clr  opc_shock_cyl=Visual.part.opc  radius_shock_cyl=Visual.Shock.cyl.rad  clr_shock_piston=Visual.Shock.piston.clr  opc_shock_piston=Visual.part.opc  clr_shock_bumpstop=Visual.Shock.bumpstop.clr  opc_shock_bumpstop=Visual.part.opc  deadvol_len_shock_cyl=Visual.Shock.dead_length  piston_len_shock=Visual.Shock.piston.len  cyl_cap_len_shock=Visual.Shock.cap.len  bumpstop_len_shock=Visual.Shock.bumpstop.len  upr_mass=Linkage.Upright.m.Value  atoe=Linkage.Upright.aToe.Value  acamber=Linkage.Upright.aCamber.Value  axle_len=Linkage.Upright.xAxle.Value  axle_whlc_to_bearing=Linkage.Upright.xWCtoBearing.Value  axle_mass=Linkage.Upright.mAxle.Value  clr_conn_upr=Visual.hp.clr  opc_conn_upr=Visual.hp.opc  size_conn_upr=Visual.hp.rad  clr_upr=Visual.Upright.clr  opc_upr=Visual.part.opc  radius_upr=Visual.Upright.rad  clr_axle=Visual.Axle.clr  opc_axle=Visual.part.opc  radius_axle=Visual.Axle.rad  rod_mass=Linkage.TrackRod.m.Value  clr_conn_rod=Visual.hp.clr  opc_conn_rod=Visual.hp.opc  size_conn_rod=Visual.hp.rad  clr_rod=Visual.TrackRod.clr  opc_rod=Visual.part.opc  radius_rod=Visual.TrackRod.rad  whl_init_spd_lr=InitLinkage.nWheel.Value
  MacPhersonSplitLowerArm : Linkage_MacPherson_SpLA/MacPhersonSplitLowerArm  VariantControl=MacPhersonSplitLowerArm  popup_leftRight=Left  hp_in_f_la=Linkage.LowerArmF.sInboard.Value  hp_in_r_la=Linkage.LowerArmR.sInboard.Value  hp_out_f_la=Linkage.LowerArmF.sOutboard.Value  hp_out_r_la=Linkage.LowerArmR.sOutboard.Value  hp_upr_cg=Linkage.Upright.sCG.Value  hp_upr_wc=Linkage.Upright.sWheelCentre.Value  hp_upr_arb=Linkage.Upright.sARB.Value  hp_in_rod=Linkage.TrackRod.sInboard.Value  hp_upr_rod=Linkage.TrackRod.sOutboard.Value  hp_spr_top=Linkage.Shock.sTop.Value  hp_spr_bot=Linkage.Shock.sBottom.Value  clr_hp=Visual.hp.clr  opc_hp=Visual.hp.opc  size_hp=Visual.hp.rad  Lower_ArmF_to_Subframe=Linkage.LowerArmF_to_Subframe  Lower_ArmR_to_Subframe=Linkage.LowerArmR_to_Subframe  LowerArmF_to_Upright=Linkage.LowerArmF_to_Upright  LowerArmR_to_Upright=Linkage.LowerArmR_to_Upright  laf_mass=Linkage.LowerArmF.m.Value  lar_mass=Linkage.LowerArmR.m.Value  clr_conn_links=Visual.hp.clr  opc_conn_links=Visual.hp.opc  size_conn_links=Visual.hp.rad  clr_laf=Visual.LowerArm.clr  opc_laf=Visual.part.opc  radius_laf=Visual.LowerArm.rad  clr_lar=Visual.LowerArm.clr  opc_lar=Visual.part.opc  radius_lar=Visual.LowerArm.rad  Shock_to_Subframe=Linkage.Shock_to_Subframe  shock_pist_mass=Linkage.Shock.mPiston.Value  shock_cyl_mass=Linkage.Shock.mCylinder.Value  up_lim_bumpstop=Linkage.Endstop.xMax.Value  low_lim_bumpstop=Linkage.Endstop.xMin.Value  clr_conn_shock=Visual.hp.clr  opc_conn_shock=Visual.hp.opc  size_conn_shock=Visual.hp.rad  clr_shock_cyl=Visual.Shock.cyl.clr  opc_shock_cyl=Visual.part.opc  radius_shock_cyl=Visual.Shock.cyl.rad  clr_shock_piston=Visual.Shock.piston.clr  opc_shock_piston=Visual.part.opc  clr_shock_bumpstop=Visual.Shock.bumpstop.clr  opc_shock_bumpstop=Visual.part.opc  deadvol_len_shock_cyl=Visual.Shock.dead_length  piston_len_shock=Visual.Shock.piston.len  cyl_cap_len_shock=Visual.Shock.cap.len  bumpstop_len_shock=Visual.Shock.bumpstop.len  upr_mass=Linkage.Upright.m.Value  atoe=Linkage.Upright.aToe.Value  acamber=Linkage.Upright.aCamber.Value  axle_len=Linkage.Upright.xAxle.Value  axle_whlc_to_bearing=Linkage.Upright.xWCtoBearing.Value  axle_mass=Linkage.Upright.mAxle.Value  clr_conn_upr=Visual.hp.clr  opc_conn_upr=Visual.hp.opc  size_conn_upr=Visual.hp.rad  clr_upr=Visual.Upright.clr  opc_upr=Visual.part.opc  radius_upr=Visual.Upright.rad  clr_axle=Visual.Axle.clr  opc_axle=Visual.part.opc  radius_axle=Visual.Axle.rad  rod_mass=Linkage.TrackRod.m.Value  clr_conn_rod=Visual.hp.clr  opc_conn_rod=Visual.hp.opc  size_conn_rod=Visual.hp.rad  clr_rod=Visual.TrackRod.clr  opc_rod=Visual.part.opc  radius_rod=Visual.TrackRod.rad  whl_init_spd_lr=InitLinkage.nWheel.Value
  SplitLowerArmShockFront : Linkage_SpLA_S2LAF/SplitLowerArmShockFront  VariantControl=SplitLowerArmShockFront  popup_leftRight=Left  hp_in_f_ua=Linkage.UpperWishbone.sInboardF.Value  hp_in_r_ua=Linkage.UpperWishbone.sInboardR.Value  hp_out_ua=Linkage.UpperWishbone.sOutboard.Value  hp_in_f_la=Linkage.LowerArmF.sInboard.Value  hp_in_r_la=Linkage.LowerArmR.sInboard.Value  hp_out_f_la=Linkage.LowerArmF.sOutboard.Value  hp_out_r_la=Linkage.LowerArmR.sOutboard.Value  hp_arb=Linkage.LowerArmR.sARB.Value  hp_upr_cg=Linkage.Upright.sCG.Value  hp_upr_wc=Linkage.Upright.sWheelCentre.Value  hp_in_rod=Linkage.TrackRod.sInboard.Value  hp_upr_rod=Linkage.TrackRod.sOutboard.Value  hp_spr_top=Linkage.Shock.sTop.Value  hp_spr_bot=Linkage.Shock.sBottom.Value  clr_hp=Visual.hp.clr  opc_hp=Visual.hp.opc  size_hp=Visual.hp.rad  Upper_Arm_to_Subframe=Linkage.Upper_Arm_to_Subframe  ua_mass=Linkage.UpperWishbone.m.Value  clr_ua=Visual.UpperArm.clr  opc_ua=Visual.part.opc  radius_ua=Visual.UpperArm.rad  LowerArmF_to_Subframe=Linkage.LowerArmF_to_Subframe  LowerArmR_to_Subframe=Linkage.LowerArmR_to_Subframe  laf_mass=Linkage.LowerArmF.m.Value  lar_mass=Linkage.LowerArmR.m.Value  clr_conn_la=Visual.hp.clr  opc_conn_la=Visual.hp.opc  size_conn_la=Visual.hp.rad  clr_laf=Visual.LowerArm.clr  opc_laf=Visual.part.opc  radius_laf=Visual.LowerArm.rad  clr_lar=Visual.LowerArm.clr  opc_lar=Visual.part.opc  radius_lar=Visual.LowerArm.rad  shock_pist_mass=Linkage.Shock.mPiston.Value  shock_cyl_mass=Linkage.Shock.mCylinder.Value  up_lim_bumpstop=Linkage.Endstop.xMax.Value  low_lim_bumpstop=Linkage.Endstop.xMin.Value  clr_conn_shock=Visual.hp.clr  opc_conn_shock=Visual.hp.opc  size_conn_shock=Visual.hp.rad  clr_shock_cyl=Visual.Shock.cyl.clr  opc_shock_cyl=Visual.part.opc  radius_shock_cyl=Visual.Shock.cyl.rad  clr_shock_piston=Visual.Shock.piston.clr  opc_shock_piston=Visual.part.opc  clr_shock_bumpstop=Visual.Shock.bumpstop.clr  opc_shock_bumpstop=Visual.part.opc  deadvol_len_shock_cyl=Visual.Shock.dead_length  piston_len_shock=Visual.Shock.piston.len  cyl_cap_len_shock=Visual.Shock.cap.len  bumpstop_len_shock=Visual.Shock.bumpstop.len  atoe=Linkage.Upright.aToe.Value  acamber=Linkage.Upright.aCamber.Value  upr_mass=Linkage.Upright.m.Value  axle_len=Linkage.Upright.xAxle.Value  axle_whlc_to_bearing=Linkage.Upright.xWCtoBearing.Value  axle_mass=Linkage.Upright.mAxle.Value  clr_conn_upr=Visual.hp.clr  opc_conn_upr=Visual.hp.opc  size_conn_upr=Visual.hp.rad  clr_upr=Visual.Upright.clr  opc_upr=Visual.part.opc  radius_upr=Visual.Upright.rad  clr_axle=Visual.Axle.clr  opc_axle=Visual.part.opc  radius_axle=Visual.Axle.rad  rod_mass=Linkage.TrackRod.m.Value  clr_conn_rod=Visual.hp.clr  opc_conn_rod=Visual.hp.opc  size_conn_rod=Visual.hp.rad  clr_rod=Visual.TrackRod.clr  opc_rod=Visual.part.opc  radius_rod=Visual.TrackRod.rad  whl_init_spd_lr=InitLinkage.nWheel.Value
  SplitLowerArmShockFrontAD : Linkage_SpLA_S2LAF_AD/SplitLowerArmShockFrontAD  VariantControl=SplitLowerArmShockFrontAD  popup_leftRight=Left  hp_in_f_ua=Linkage.UpperWishbone.sInboardF.Value  hp_in_r_ua=Linkage.UpperWishbone.sInboardR.Value  hp_out_ua=Linkage.UpperWishbone.sOutboard.Value  hp_in_f_la=Linkage.LowerArmF.sInboard.Value  hp_in_r_la=Linkage.LowerArmR.sInboard.Value  hp_out_f_la=Linkage.LowerArmF.sOutboard.Value  hp_out_r_la=Linkage.LowerArmR.sOutboard.Value  hp_arb=Linkage.Shock.sARB.Value  hp_upr_cg=Linkage.Upright.sCG.Value  hp_upr_wc=Linkage.Upright.sWheelCentre.Value  hp_in_rod=Linkage.TrackRod.sInboard.Value  hp_upr_rod=Linkage.TrackRod.sOutboard.Value  hp_spr_top=Linkage.Shock.sTop.Value  hp_spr_bot=Linkage.Shock.sBottom.Value  clr_hp=Visual.hp.clr  opc_hp=Visual.hp.opc  size_hp=Visual.hp.rad  Upper_Arm_to_Subframe=Linkage.Upper_Arm_to_Subframe  ua_mass=Linkage.UpperWishbone.m.Value  clr_ua=Visual.UpperArm.clr  opc_ua=Visual.part.opc  radius_ua=Visual.UpperArm.rad  LowerArmF_to_Subframe=Linkage.LowerArmF_to_Subframe  LowerArmR_to_Subframe=Linkage.LowerArmR_to_Subframe  laf_mass=Linkage.LowerArmF.m.Value  lar_mass=Linkage.LowerArmR.m.Value  clr_conn_la=Visual.hp.clr  opc_conn_la=Visual.hp.opc  size_conn_la=Visual.hp.rad  clr_laf=Visual.LowerArm.clr  opc_laf=Visual.part.opc  radius_laf=Visual.LowerArm.rad  clr_lar=Visual.LowerArm.clr  opc_lar=Visual.part.opc  radius_lar=Visual.LowerArm.rad  shock_pist_mass=Linkage.Shock.mPiston.Value  shock_cyl_mass=Linkage.Shock.mCylinder.Value  up_lim_bumpstop=Linkage.Endstop.xMax.Value  low_lim_bumpstop=Linkage.Endstop.xMin.Value  clr_conn_shock=Visual.hp.clr  opc_conn_shock=Visual.hp.opc  size_conn_shock=Visual.hp.rad  clr_shock_cyl=Visual.Shock.cyl.clr  opc_shock_cyl=Visual.part.opc  radius_shock_cyl=Visual.Shock.cyl.rad  clr_shock_piston=Visual.Shock.piston.clr  opc_shock_piston=Visual.part.opc  clr_shock_bumpstop=Visual.Shock.bumpstop.clr  opc_shock_bumpstop=Visual.part.opc  deadvol_len_shock_cyl=Visual.Shock.dead_length  piston_len_shock=Visual.Shock.piston.len  cyl_cap_len_shock=Visual.Shock.cap.len  bumpstop_len_shock=Visual.Shock.bumpstop.len  atoe=Linkage.Upright.aToe.Value  acamber=Linkage.Upright.aCamber.Value  upr_mass=Linkage.Upright.m.Value  axle_len=Linkage.Upright.xAxle.Value  axle_whlc_to_bearing=Linkage.Upright.xWCtoBearing.Value  axle_mass=Linkage.Upright.mAxle.Value  clr_conn_upr=Visual.hp.clr  opc_conn_upr=Visual.hp.opc  size_conn_upr=Visual.hp.rad  clr_upr=Visual.Upright.clr  opc_upr=Visual.part.opc  radius_upr=Visual.Upright.rad  clr_axle=Visual.Axle.clr  opc_axle=Visual.part.opc  radius_axle=Visual.Axle.rad  rod_mass=Linkage.TrackRod.m.Value  clr_conn_rod=Visual.hp.clr  opc_conn_rod=Visual.hp.opc  size_conn_rod=Visual.hp.rad  clr_rod=Visual.TrackRod.clr  opc_rod=Visual.part.opc  radius_rod=Visual.TrackRod.rad  whl_init_spd_lr=InitLinkage.nWheel.Value
  SplitLowerArmShockFrontAU : Linkage_SpLA_S2LAF_AU/SplitLowerArmShockFrontAU  VariantControl=SplitLowerArmShockFrontAU  popup_leftRight=Left  hp_in_f_ua=Linkage.UpperWishbone.sInboardF.Value  hp_in_r_ua=Linkage.UpperWishbone.sInboardR.Value  hp_out_ua=Linkage.UpperWishbone.sOutboard.Value  hp_in_f_la=Linkage.LowerArmF.sInboard.Value  hp_in_r_la=Linkage.LowerArmR.sInboard.Value  hp_out_f_la=Linkage.LowerArmF.sOutboard.Value  hp_out_r_la=Linkage.LowerArmR.sOutboard.Value  hp_upr_cg=Linkage.Upright.sCG.Value  hp_upr_wc=Linkage.Upright.sWheelCentre.Value  hp_upr_arb=Linkage.Upright.sARB.Value  hp_in_rod=Linkage.TrackRod.sInboard.Value  hp_upr_rod=Linkage.TrackRod.sOutboard.Value  hp_spr_top=Linkage.Shock.sTop.Value  hp_spr_bot=Linkage.Shock.sBottom.Value  clr_hp=Visual.hp.clr  opc_hp=Visual.hp.opc  size_hp=Visual.hp.rad  Upper_Arm_to_Subframe=Linkage.Upper_Arm_to_Subframe  ua_mass=Linkage.UpperWishbone.m.Value  clr_ua=Visual.UpperArm.clr  opc_ua=Visual.part.opc  radius_ua=Visual.UpperArm.rad  LowerArmF_to_Subframe=Linkage.LowerArmF_to_Subframe  LowerArmR_to_Subframe=Linkage.LowerArmR_to_Subframe  laf_mass=Linkage.LowerArmF.m.Value  lar_mass=Linkage.LowerArmR.m.Value  clr_conn_la=Visual.hp.clr  opc_conn_la=Visual.hp.opc  size_conn_la=Visual.hp.rad  clr_laf=Visual.LowerArm.clr  opc_laf=Visual.part.opc  radius_laf=Visual.LowerArm.rad  clr_lar=Visual.LowerArm.clr  opc_lar=Visual.part.opc  radius_lar=Visual.LowerArm.rad  shock_pist_mass=Linkage.Shock.mPiston.Value  shock_cyl_mass=Linkage.Shock.mCylinder.Value  up_lim_bumpstop=Linkage.Endstop.xMax.Value  low_lim_bumpstop=Linkage.Endstop.xMin.Value  clr_conn_shock=Visual.hp.clr  opc_conn_shock=Visual.hp.opc  size_conn_shock=Visual.hp.rad  clr_shock_cyl=Visual.Shock.cyl.clr  opc_shock_cyl=Visual.part.opc  radius_shock_cyl=Visual.Shock.cyl.rad  clr_shock_piston=Visual.Shock.piston.clr  opc_shock_piston=Visual.part.opc  clr_shock_bumpstop=Visual.Shock.bumpstop.clr  opc_shock_bumpstop=Visual.part.opc  deadvol_len_shock_cyl=Visual.Shock.dead_length  piston_len_shock=Visual.Shock.piston.len  cyl_cap_len_shock=Visual.Shock.cap.len  bumpstop_len_shock=Visual.Shock.bumpstop.len  atoe=Linkage.Upright.aToe.Value  acamber=Linkage.Upright.aCamber.Value  upr_mass=Linkage.Upright.m.Value  axle_len=Linkage.Upright.xAxle.Value  axle_whlc_to_bearing=Linkage.Upright.xWCtoBearing.Value  axle_mass=Linkage.Upright.mAxle.Value  clr_conn_upr=Visual.hp.clr  opc_conn_upr=Visual.hp.opc  size_conn_upr=Visual.hp.rad  clr_upr=Visual.Upright.clr  opc_upr=Visual.part.opc  radius_upr=Visual.Upright.rad  clr_axle=Visual.Axle.clr  opc_axle=Visual.part.opc  radius_axle=Visual.Axle.rad  rod_mass=Linkage.TrackRod.m.Value  clr_conn_rod=Visual.hp.clr  opc_conn_rod=Visual.hp.opc  size_conn_rod=Visual.hp.rad  clr_rod=Visual.TrackRod.clr  opc_rod=Visual.part.opc  radius_rod=Visual.TrackRod.rad  whl_init_spd_lr=InitLinkage.nWheel.Value
  SplitLowerArmShockRear : Linkage_SpLA_S2LAR/SplitLowerArmShockRear  VariantControl=SplitLowerArmShockRear  popup_leftRight=Left  hp_in_f_ua=Linkage.UpperWishbone.sInboardF.Value  hp_in_r_ua=Linkage.UpperWishbone.sInboardR.Value  hp_out_ua=Linkage.UpperWishbone.sOutboard.Value  hp_in_f_la=Linkage.LowerArmF.sInboard.Value  hp_in_r_la=Linkage.LowerArmR.sInboard.Value  hp_out_f_la=Linkage.LowerArmF.sOutboard.Value  hp_out_r_la=Linkage.LowerArmR.sOutboard.Value  hp_arb=Linkage.LowerArmR.sARB.Value  hp_upr_cg=Linkage.Upright.sCG.Value  hp_upr_wc=Linkage.Upright.sWheelCentre.Value  hp_in_rod=Linkage.TrackRod.sInboard.Value  hp_upr_rod=Linkage.TrackRod.sOutboard.Value  hp_spr_top=Linkage.Shock.sTop.Value  hp_spr_bot=Linkage.Shock.sBottom.Value  clr_hp=Visual.hp.clr  opc_hp=Visual.hp.opc  size_hp=Visual.hp.rad  Upper_Arm_to_Subframe=Linkage.Upper_Arm_to_Subframe  ua_mass=Linkage.UpperWishbone.m.Value  clr_ua=Visual.UpperArm.clr  opc_ua=Visual.part.opc  radius_ua=Visual.UpperArm.rad  LowerArmF_to_Subframe=Linkage.LowerArmF_to_Subframe  LowerArmR_to_Subframe=Linkage.LowerArmR_to_Subframe  laf_mass=Linkage.LowerArmF.m.Value  lar_mass=Linkage.LowerArmR.m.Value  clr_conn_la=Visual.hp.clr  opc_conn_la=Visual.hp.opc  size_conn_la=Visual.hp.rad  clr_laf=Visual.LowerArm.clr  opc_laf=Visual.part.opc  radius_laf=Visual.LowerArm.rad  clr_lar=Visual.LowerArm.clr  opc_lar=Visual.part.opc  radius_lar=Visual.LowerArm.rad  shock_pist_mass=Linkage.Shock.mPiston.Value  shock_cyl_mass=Linkage.Shock.mCylinder.Value  up_lim_bumpstop=Linkage.Endstop.xMax.Value  low_lim_bumpstop=Linkage.Endstop.xMin.Value  clr_conn_shock=Visual.hp.clr  opc_conn_shock=Visual.hp.opc  size_conn_shock=Visual.hp.rad  clr_shock_cyl=Visual.Shock.cyl.clr  opc_shock_cyl=Visual.part.opc  radius_shock_cyl=Visual.Shock.cyl.rad  clr_shock_piston=Visual.Shock.piston.clr  opc_shock_piston=Visual.part.opc  clr_shock_bumpstop=Visual.Shock.bumpstop.clr  opc_shock_bumpstop=Visual.part.opc  deadvol_len_shock_cyl=Visual.Shock.dead_length  piston_len_shock=Visual.Shock.piston.len  cyl_cap_len_shock=Visual.Shock.cap.len  bumpstop_len_shock=Visual.Shock.bumpstop.len  atoe=Linkage.Upright.aToe.Value  acamber=Linkage.Upright.aCamber.Value  upr_mass=Linkage.Upright.m.Value  axle_len=Linkage.Upright.xAxle.Value  axle_whlc_to_bearing=Linkage.Upright.xWCtoBearing.Value  axle_mass=Linkage.Upright.mAxle.Value  clr_conn_upr=Visual.hp.clr  opc_conn_upr=Visual.hp.opc  size_conn_upr=Visual.hp.rad  clr_upr=Visual.Upright.clr  opc_upr=Visual.part.opc  radius_upr=Visual.Upright.rad  clr_axle=Visual.Axle.clr  opc_axle=Visual.part.opc  radius_axle=Visual.Axle.rad  rod_mass=Linkage.TrackRod.m.Value  clr_conn_rod=Visual.hp.clr  opc_conn_rod=Visual.hp.opc  size_conn_rod=Visual.hp.rad  clr_rod=Visual.TrackRod.clr  opc_rod=Visual.part.opc  radius_rod=Visual.TrackRod.rad  whl_init_spd_lr=InitLinkage.nWheel.Value
  SplitLowerArmShockRearAD : Linkage_SpLA_S2LAR_AD/SplitLowerArmShockRearAD  VariantControl=SplitLowerArmShockRearAD  popup_leftRight=Left  hp_in_f_ua=Linkage.UpperWishbone.sInboardF.Value  hp_in_r_ua=Linkage.UpperWishbone.sInboardR.Value  hp_out_ua=Linkage.UpperWishbone.sOutboard.Value  hp_in_f_la=Linkage.LowerArmF.sInboard.Value  hp_in_r_la=Linkage.LowerArmR.sInboard.Value  hp_out_f_la=Linkage.LowerArmF.sOutboard.Value  hp_out_r_la=Linkage.LowerArmR.sOutboard.Value  hp_arb=Linkage.Shock.sARB.Value  hp_upr_cg=Linkage.Upright.sCG.Value  hp_upr_wc=Linkage.Upright.sWheelCentre.Value  hp_in_rod=Linkage.TrackRod.sInboard.Value  hp_upr_rod=Linkage.TrackRod.sOutboard.Value  hp_spr_top=Linkage.Shock.sTop.Value  hp_spr_bot=Linkage.Shock.sBottom.Value  clr_hp=Visual.hp.clr  opc_hp=Visual.hp.opc  size_hp=Visual.hp.rad  Upper_Arm_to_Subframe=Linkage.Upper_Arm_to_Subframe  ua_mass=Linkage.UpperWishbone.m.Value  clr_ua=Visual.UpperArm.clr  opc_ua=Visual.part.opc  radius_ua=Visual.UpperArm.rad  LowerArmF_to_Subframe=Linkage.LowerArmF_to_Subframe  LowerArmR_to_Subframe=Linkage.LowerArmR_to_Subframe  laf_mass=Linkage.LowerArmF.m.Value  lar_mass=Linkage.LowerArmR.m.Value  clr_conn_la=Visual.hp.clr  opc_conn_la=Visual.hp.opc  size_conn_la=Visual.hp.rad  clr_laf=Visual.LowerArm.clr  opc_laf=Visual.part.opc  radius_laf=Visual.LowerArm.rad  clr_lar=Visual.LowerArm.clr  opc_lar=Visual.part.opc  radius_lar=Visual.LowerArm.rad  shock_pist_mass=Linkage.Shock.mPiston.Value  shock_cyl_mass=Linkage.Shock.mCylinder.Value  up_lim_bumpstop=Linkage.Endstop.xMax.Value  low_lim_bumpstop=Linkage.Endstop.xMin.Value  clr_conn_shock=Visual.hp.clr  opc_conn_shock=Visual.hp.opc  size_conn_shock=Visual.hp.rad  clr_shock_cyl=Visual.Shock.cyl.clr  opc_shock_cyl=Visual.part.opc  radius_shock_cyl=Visual.Shock.cyl.rad  clr_shock_piston=Visual.Shock.piston.clr  opc_shock_piston=Visual.part.opc  clr_shock_bumpstop=Visual.Shock.bumpstop.clr  opc_shock_bumpstop=Visual.part.opc  deadvol_len_shock_cyl=Visual.Shock.dead_length  piston_len_shock=Visual.Shock.piston.len  cyl_cap_len_shock=Visual.Shock.cap.len  bumpstop_len_shock=Visual.Shock.bumpstop.len  atoe=Linkage.Upright.aToe.Value  acamber=Linkage.Upright.aCamber.Value  upr_mass=Linkage.Upright.m.Value  axle_len=Linkage.Upright.xAxle.Value  axle_whlc_to_bearing=Linkage.Upright.xWCtoBearing.Value  axle_mass=Linkage.Upright.mAxle.Value  clr_conn_upr=Visual.hp.clr  opc_conn_upr=Visual.hp.opc  size_conn_upr=Visual.hp.rad  clr_upr=Visual.Upright.clr  opc_upr=Visual.part.opc  radius_upr=Visual.Upright.rad  clr_axle=Visual.Axle.clr  opc_axle=Visual.part.opc  radius_axle=Visual.Axle.rad  rod_mass=Linkage.TrackRod.m.Value  clr_conn_rod=Visual.hp.clr  opc_conn_rod=Visual.hp.opc  size_conn_rod=Visual.hp.rad  clr_rod=Visual.TrackRod.clr  opc_rod=Visual.part.opc  radius_rod=Visual.TrackRod.rad  whl_init_spd_lr=InitLinkage.nWheel.Value
  SplitLowerArmShockRearAU : Linkage_SpLA_S2LAR_AU/SplitLowerArmShockRearAU  VariantControl=SplitLowerArmShockRearAU  popup_leftRight=Left  hp_in_f_ua=Linkage.UpperWishbone.sInboardF.Value  hp_in_r_ua=Linkage.UpperWishbone.sInboardR.Value  hp_out_ua=Linkage.UpperWishbone.sOutboard.Value  hp_in_f_la=Linkage.LowerArmF.sInboard.Value  hp_in_r_la=Linkage.LowerArmR.sInboard.Value  hp_out_f_la=Linkage.LowerArmF.sOutboard.Value  hp_out_r_la=Linkage.LowerArmR.sOutboard.Value  hp_upr_cg=Linkage.Upright.sCG.Value  hp_upr_wc=Linkage.Upright.sWheelCentre.Value  hp_upr_arb=Linkage.Upright.sARB.Value  hp_in_rod=Linkage.TrackRod.sInboard.Value  hp_upr_rod=Linkage.TrackRod.sOutboard.Value  hp_spr_top=Linkage.Shock.sTop.Value  hp_spr_bot=Linkage.Shock.sBottom.Value  clr_hp=Visual.hp.clr  opc_hp=Visual.hp.opc  size_hp=Visual.hp.rad  Upper_Arm_to_Subframe=Linkage.Upper_Arm_to_Subframe  ua_mass=Linkage.UpperWishbone.m.Value  clr_ua=Visual.UpperArm.clr  opc_ua=Visual.part.opc  radius_ua=Visual.UpperArm.rad  LowerArmF_to_Subframe=Linkage.LowerArmF_to_Subframe  LowerArmR_to_Subframe=Linkage.LowerArmR_to_Subframe  laf_mass=Linkage.LowerArmF.m.Value  lar_mass=Linkage.LowerArmR.m.Value  clr_conn_la=Visual.hp.clr  opc_conn_la=Visual.hp.opc  size_conn_la=Visual.hp.rad  clr_laf=Visual.LowerArm.clr  opc_laf=Visual.part.opc  radius_laf=Visual.LowerArm.rad  clr_lar=Visual.LowerArm.clr  opc_lar=Visual.part.opc  radius_lar=Visual.LowerArm.rad  shock_pist_mass=Linkage.Shock.mPiston.Value  shock_cyl_mass=Linkage.Shock.mCylinder.Value  up_lim_bumpstop=Linkage.Endstop.xMax.Value  low_lim_bumpstop=Linkage.Endstop.xMin.Value  clr_conn_shock=Visual.hp.clr  opc_conn_shock=Visual.hp.opc  size_conn_shock=Visual.hp.rad  clr_shock_cyl=Visual.Shock.cyl.clr  opc_shock_cyl=Visual.part.opc  radius_shock_cyl=Visual.Shock.cyl.rad  clr_shock_piston=Visual.Shock.piston.clr  opc_shock_piston=Visual.part.opc  clr_shock_bumpstop=Visual.Shock.bumpstop.clr  opc_shock_bumpstop=Visual.part.opc  deadvol_len_shock_cyl=Visual.Shock.dead_length  piston_len_shock=Visual.Shock.piston.len  cyl_cap_len_shock=Visual.Shock.cap.len  bumpstop_len_shock=Visual.Shock.bumpstop.len  atoe=Linkage.Upright.aToe.Value  acamber=Linkage.Upright.aCamber.Value  upr_mass=Linkage.Upright.m.Value  axle_len=Linkage.Upright.xAxle.Value  axle_whlc_to_bearing=Linkage.Upright.xWCtoBearing.Value  axle_mass=Linkage.Upright.mAxle.Value  clr_conn_upr=Visual.hp.clr  opc_conn_upr=Visual.hp.opc  size_conn_upr=Visual.hp.rad  clr_upr=Visual.Upright.clr  opc_upr=Visual.part.opc  radius_upr=Visual.Upright.rad  clr_axle=Visual.Axle.clr  opc_axle=Visual.part.opc  radius_axle=Visual.Axle.rad  rod_mass=Linkage.TrackRod.m.Value  clr_conn_rod=Visual.hp.clr  opc_conn_rod=Visual.hp.opc  size_conn_rod=Visual.hp.rad  clr_rod=Visual.TrackRod.clr  opc_rod=Visual.part.opc  radius_rod=Visual.TrackRod.rad  whl_init_spd_lr=InitLinkage.nWheel.Value
  Rack : PMIOPort  Side=Right
  Ref : PMIOPort  Port=2  Side=Right
  WhlC : PMIOPort  Port=3  Side=Left
  RaceSpin : PMIOPort  Port=4  Side=Left
  RaceFix : PMIOPort  Port=5  Side=Left
  Axle1D : PMIOPort  Port=6  Side=Left
  AxleIn : PMIOPort  Port=7  Side=Left
  S : PMIOPort  Port=8  Side=Left
  D : PMIOPort  Port=9  Side=Left
  AR : PMIOPort  Port=10  Side=Left
  m : Outport  VectorParamsAs1DForOutWhenUnconnected=off
